simulink subsystem "IR_LED_Pattern"  (R2024a)
settings: Solver=VariableStepAuto  StartTime=0.0  StopTime=10.0  RelTol=1e-3
undefined symbols (not defined in the file): IR_LED_PERIOD
libraries: simulink_extras x1
settings Model: Creator=JesseJabezArendse  LastModifiedBy=zaino
settings RTWCC: GPUComputeCapability=3.5

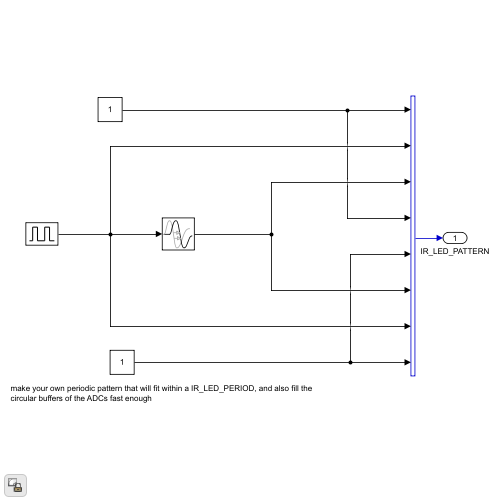
[thumbnail: Simulink's stored preview of the top-level diagram]
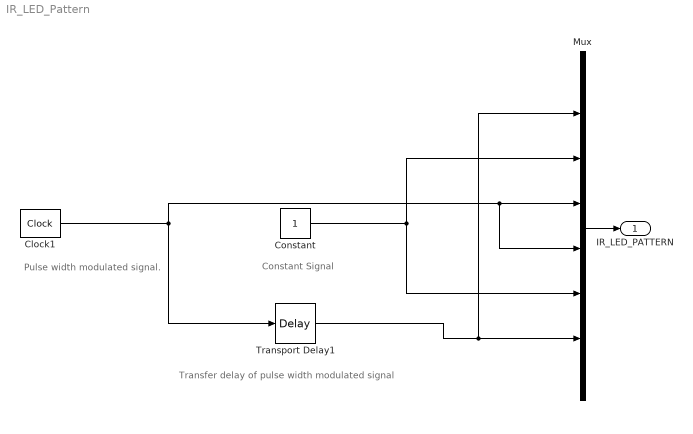
== system IR_LED_Pattern ==
  note: Transfer delay of pulse width modulated signal
  note: Pulse width modulated signal.
  note: Constant Signal
  Clock1 : simulink_extras/Flip Flops/Clock  period=IR_LED_PERIOD
  Constant : Constant
  Mux : Mux  Inputs=8
  Transport Delay1 : TransportDelay  DelayTime=0.5*IR_LED_PERIOD
  IR_LED_PATTERN : Outport
  wires:
  Mux/1 -> IR_LED_PATTERN/1
  Constant/1 -> Mux/3, Mux/6
  Transport Delay1/1 -> Mux/7, Mux/2
  Clock1/1 -> Mux/4, Mux/5, Transport Delay1/1
